simulink model "bf_4x"  (R2013a)
settings: Solver=VariableStepDiscrete  StartTime=0.0  StopTime=1000  RelTol=1e-3
undefined symbols (not defined in the file): enable, misc_lib, pfb_coeff_gen_calc
libraries: xbsIndex_r4 x6358, casper_library_misc x119, casper_library_delays x24, casper_library_multipliers x20, simulink x16, casper_library_pfbs x4, xbsReplacements_r4 x2, xps_library x1
(part 6 of 73)

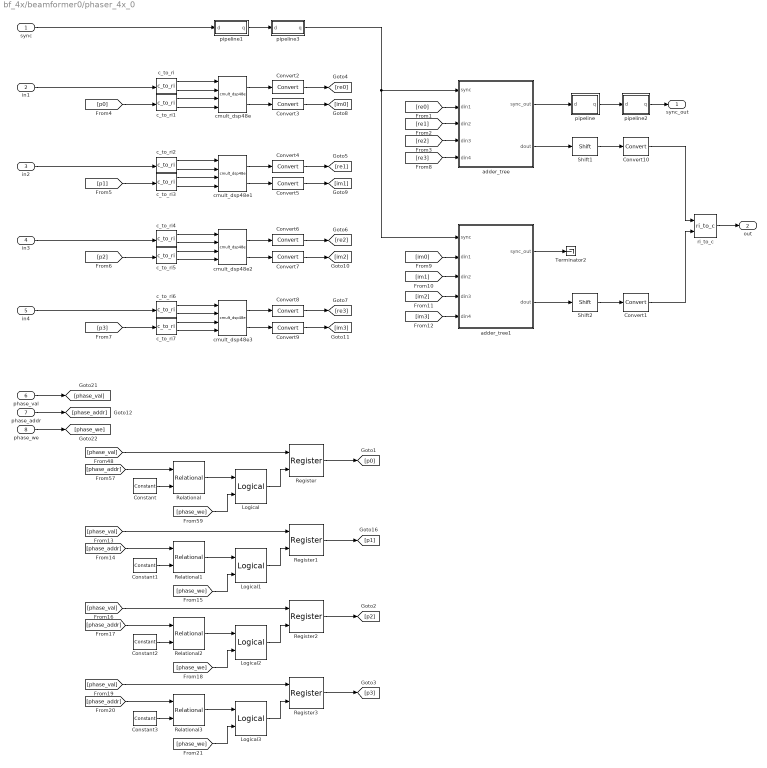
== system bf_4x/beamformer0/phaser_4x_0 ==
  sync : Inport
  in1 : Inport  Port=2
  in2 : Inport  Port=3
  in3 : Inport  Port=4
  in4 : Inport  Port=5
  phase_val : Inport  Port=6
  phase_addr : Inport  Port=7
  phase_we : Inport  Port=8
  Constant : xbsIndex_r4/Constant  const=sub_addr(1)  gui_display_data_type=Fixed-point  arith_type=Unsigned  n_bits=32  bin_pt=0  preci_type=Single  exp_width=8  frac_width=24  explicit_period=on  period=1  equ=P=C  opselect=C  inp2=PCIN>>17  opr=+  inp1=P  carry=CIN  dbl_ovrd=off  block_type=constant
  Constant1 : xbsIndex_r4/Constant  const=sub_addr(2)  gui_display_data_type=Fixed-point  arith_type=Unsigned  n_bits=32  bin_pt=0  preci_type=Single  exp_width=8  frac_width=24  explicit_period=on  period=1  equ=P=C  opselect=C  inp2=PCIN>>17  opr=+  inp1=P  carry=CIN  dbl_ovrd=off  block_type=constant
  Constant2 : xbsIndex_r4/Constant  const=sub_addr(3)  gui_display_data_type=Fixed-point  arith_type=Unsigned  n_bits=32  bin_pt=0  preci_type=Single  exp_width=8  frac_width=24  explicit_period=on  period=1  equ=P=C  opselect=C  inp2=PCIN>>17  opr=+  inp1=P  carry=CIN  dbl_ovrd=off  block_type=constant
  Constant3 : xbsIndex_r4/Constant  const=sub_addr(4)  gui_display_data_type=Fixed-point  arith_type=Unsigned  n_bits=32  bin_pt=0  preci_type=Single  exp_width=8  frac_width=24  explicit_period=on  period=1  equ=P=C  opselect=C  inp2=PCIN>>17  opr=+  inp1=P  carry=CIN  dbl_ovrd=off  block_type=constant
  Convert{1..10} (10 alike) : xbsIndex_r4/Convert  gui_display_data_type=Fixed-point  arith_type=Unsigned  n_bits=18  bin_pt=17  float_type=Single  exp_bits=8  fraction_bits=24  quantization=Truncate  overflow=Wrap  en=off  latency=2  dbl_ovrd=off  pipeline=off  block_type=convert
      settings: block_version=11.4
  Logical{,1..3} (4 alike) : xbsIndex_r4/Logical  logical_function=AND  inputs=2  en=off  latency=0  precision=Full  arith_type=Unsigned  n_bits=16  bin_pt=0  align_bp=on  dbl_ovrd=off  block_type=logical
  Register{,1..3} (4 alike) : xbsIndex_r4/Register  init=0  rst=off  en=on  dbl_ovrd=off  block_type=register
  Relational{,1..3} (4 alike) : xbsIndex_r4/Relational  mode=a=b  en=off  latency=0  dbl_ovrd=off  block_type=relational
  Shift1 : xbsIndex_r4/Shift  shift_dir=Right  shift_bits=2  en=off  latency=1  precision=Full  arith_type="Signed  (2's comp)"  n_bits=16  bin_pt=14  quantization=Truncate  overflow=Wrap  dbl_ovrd=off  block_type=shift
  Shift2 : xbsIndex_r4/Shift  shift_dir=Right  shift_bits=2  en=off  latency=1  precision=Full  arith_type="Signed  (2's comp)"  n_bits=16  bin_pt=14  quantization=Truncate  overflow=Wrap  dbl_ovrd=off  block_type=shift
  Terminator2 : Terminator
  adder_tree : Subsystem  AncestorBlock=casper_library_misc/adder_tree  mask(adder_tree){n_inputs=4, latency=1, adder_imp=Fabric, first_stage_hdl=on}
      mask prompts: n_inputs "Number of Inputs"; latency "Add Latency"; adder_imp "Adder implementation"; first_stage_hdl "Use behavioural HDL for first stage of adders"
      mask help:
      | Sums all inputs using a tree of adds and delays.
      |
      | Number of inputs: The number of inputs to the block to be summed
      | Add latency: The number of clock cycles to perform one addition (affects timing)..
      | Adder implementation: choice of fabric or DSP48E core, or behavioral HDL
      | Use behavioural HDL for first stage of adders: Causes the first stage of adders to be absorbed into DSP blocks if multipliers precede them (Virtex 5). Overrides Adder implementation
      mask init:
      | adder_tree_init(gcb, ...
      |     'n_inputs', n_inputs, ...
      |     'latency', latency, ...
      |     'adder_imp', adder_imp, ...
      |     'first_stage_hdl', first_stage_hdl);
      settings: AttributesFormatString=latency 2
      mask Help: eval('xlWeb(''http://casper.berkeley.edu/wiki/Adder_tree'')')
      mask TypeOptions adder_imp: Behavioral | Fabric | DSP48
  adder_tree1 : Subsystem  AncestorBlock=casper_library_misc/adder_tree  mask(adder_tree){n_inputs=4, latency=1, adder_imp=Fabric, first_stage_hdl=on}
      mask prompts: n_inputs "Number of Inputs"; latency "Add Latency"; adder_imp "Adder implementation"; first_stage_hdl "Use behavioural HDL for first stage of adders"
      mask help:
      | Sums all inputs using a tree of adds and delays.
      |
      | Number of inputs: The number of inputs to the block to be summed
      | Add latency: The number of clock cycles to perform one addition (affects timing)..
      | Adder implementation: choice of fabric or DSP48E core, or behavioral HDL
      | Use behavioural HDL for first stage of adders: Causes the first stage of adders to be absorbed into DSP blocks if multipliers precede them (Virtex 5). Overrides Adder implementation
      mask init:
      | adder_tree_init(gcb, ...
      |     'n_inputs', n_inputs, ...
      |     'latency', latency, ...
      |     'adder_imp', adder_imp, ...
      |     'first_stage_hdl', first_stage_hdl);
      settings: AttributesFormatString=latency 2
      mask Help: eval('xlWeb(''http://casper.berkeley.edu/wiki/Adder_tree'')')
      mask TypeOptions adder_imp: Behavioral | Fabric | DSP48
  c_to_ri{,1..7} (8 alike) : casper_library_misc/c_to_ri  n_bits=18  bin_pt=17
  cmult_dsp48e{,1..3} (4 alike) : casper_library_multipliers/cmult_dsp48e  n_bits_a=18  bin_pt_a=17  n_bits_b=18  bin_pt_b=17  conjugated=off  full_precision=on  n_bits_c=37  bin_pt_c=34  quantization=Truncate  overflow=Wrap  cast_latency=0
      settings: AttributesFormatString=|
      | 18_17 * 18_17 ==> 37_34
      | Latency=4
  pipeline : Subsystem  AncestorBlock=casper_library_delays/pipeline  mask(pipeline){latency=2}
      mask help:
      | An explicitly laid-out delay line to avoid mapping to SRL16s
      | for use in pipelining to help achieve timing closure.
      mask init:
      | pipeline_init(gcb,'latency',latency);
      settings: AttributesFormatString=Latency = %<latency>
      mask Display:
      | port_label('input', 1, 'd');
      | port_label('output', 1, 'q');
      | disp(['Z^-', num2str(latency)]);
  pipeline1 : Subsystem  AncestorBlock=casper_library_delays/pipeline  mask(pipeline){latency=4}
      mask help:
      | An explicitly laid-out delay line to avoid mapping to SRL16s
      | for use in pipelining to help achieve timing closure.
      mask init:
      | pipeline_init(gcb,'latency',latency);
      settings: AttributesFormatString=Latency = %<latency>
      mask Display:
      | port_label('input', 1, 'd');
      | port_label('output', 1, 'q');
      | disp(['Z^-', num2str(latency)]);
  pipeline2 : Subsystem  AncestorBlock=casper_library_delays/pipeline  mask(pipeline){latency=2}
      mask help:
      | An explicitly laid-out delay line to avoid mapping to SRL16s
      | for use in pipelining to help achieve timing closure.
      mask init:
      | pipeline_init(gcb,'latency',latency);
      settings: AttributesFormatString=Latency = %<latency>
      mask Display:
      | port_label('input', 1, 'd');
      | port_label('output', 1, 'q');
      | disp(['Z^-', num2str(latency)]);
  pipeline3 : Subsystem  AncestorBlock=casper_library_delays/pipeline  mask(pipeline){latency=2}
      mask help:
      | An explicitly laid-out delay line to avoid mapping to SRL16s
      | for use in pipelining to help achieve timing closure.
      mask init:
      | pipeline_init(gcb,'latency',latency);
      settings: AttributesFormatString=Latency = %<latency>
      mask Display:
      | port_label('input', 1, 'd');
      | port_label('output', 1, 'q');
      | disp(['Z^-', num2str(latency)]);
  ri_to_c : casper_library_misc/ri_to_c
  sync_out : Outport
  out : Outport  Port=2
  wires:
  phase_addr/1 -> [phase_addr]
  phase_we/1 -> [phase_we]
  [p1] -> c_to_ri3/1
  phase_val/1 -> [phase_val]
  c_to_ri3/1 -> cmult_dsp48e1/3
  Convert7/1 -> [im2]
  c_to_ri5/2 -> cmult_dsp48e2/4
  c_to_ri4/1 -> cmult_dsp48e2/1
  cmult_dsp48e2/2 -> Convert7/1
  Convert6/1 -> [re2]
  cmult_dsp48e2/1 -> Convert6/1
  [p2] -> c_to_ri5/1
  in3/1 -> c_to_ri4/1
  c_to_ri4/2 -> cmult_dsp48e2/2
  c_to_ri5/1 -> cmult_dsp48e2/3
  Convert9/1 -> [im3]
  c_to_ri7/2 -> cmult_dsp48e3/4
  c_to_ri6/1 -> cmult_dsp48e3/1
  cmult_dsp48e3/2 -> Convert9/1
  Convert8/1 -> [re3]
  cmult_dsp48e3/1 -> Convert8/1
  [p3] -> c_to_ri7/1
  in4/1 -> c_to_ri6/1
  c_to_ri6/2 -> cmult_dsp48e3/2
  c_to_ri7/1 -> cmult_dsp48e3/3
  sync/1 -> pipeline1/1(d)
  pipeline1/1(q) -> pipeline3/1(d)
  Convert3/1 -> [im0]
  c_to_ri1/2 -> cmult_dsp48e/4
  c_to_ri/1 -> cmult_dsp48e/1
  cmult_dsp48e/2 -> Convert3/1
  Convert2/1 -> [re0]
  cmult_dsp48e/1 -> Convert2/1
  [p0] -> c_to_ri1/1
  in1/1 -> c_to_ri/1
  c_to_ri/2 -> cmult_dsp48e/2
  c_to_ri1/1 -> cmult_dsp48e/3
  Convert5/1 -> [im1]
  c_to_ri3/2 -> cmult_dsp48e1/4
  c_to_ri2/1 -> cmult_dsp48e1/1
  cmult_dsp48e1/2 -> Convert5/1
  Convert4/1 -> [re1]
  cmult_dsp48e1/1 -> Convert4/1
  in2/1 -> c_to_ri2/1
  c_to_ri2/2 -> cmult_dsp48e1/2
  pipeline3/1(q) -> adder_tree1/1(sync), adder_tree/1(sync)
  adder_tree/2(dout) -> Shift1/1
  adder_tree1/2(dout) -> Shift2/1
  adder_tree/1(sync_out) -> pipeline/1(d)
  [re3] -> adder_tree/5(din4)
  [re2] -> adder_tree/4(din3)
  [re1] -> adder_tree/3(din2)
  [re0] -> adder_tree/2(din1)
  [im0] -> adder_tree1/2(din1)
  [im1] -> adder_tree1/3(din2)
  [im3] -> adder_tree1/5(din4)
  [im2] -> adder_tree1/4(din3)
  adder_tree1/1(sync_out) -> Terminator2/1
  Logical/1 -> Register/2
  Register/1 -> [p0]
  Constant/1 -> Relational/2
  Relational/1 -> Logical/1
  [phase_val] -> Register/1
  [phase_addr] -> Relational/1
  [phase_we] -> Logical/2
  Logical1/1 -> Register1/2
  Register1/1 -> [p1]
  Constant1/1 -> Relational1/2
  Relational1/1 -> Logical1/1
  [phase_val] -> Register1/1
  [phase_addr] -> Relational1/1
  [phase_we] -> Logical1/2
  Logical2/1 -> Register2/2
  Register2/1 -> [p2]
  Constant2/1 -> Relational2/2
  Relational2/1 -> Logical2/1
  [phase_val] -> Register2/1
  [phase_addr] -> Relational2/1
  [phase_we] -> Logical2/2
  Logical3/1 -> Register3/2
  Register3/1 -> [p3]
  Constant3/1 -> Relational3/2
  Relational3/1 -> Logical3/1
  [phase_val] -> Register3/1
  [phase_addr] -> Relational3/1
  [phase_we] -> Logical3/2
  pipeline/1(q) -> pipeline2/1(d)
  Shift1/1 -> Convert10/1
  Shift2/1 -> Convert1/1
  Convert1/1 -> ri_to_c/2
  Convert10/1 -> ri_to_c/1
  pipeline2/1(q) -> sync_out/1
  ri_to_c/1 -> out/1

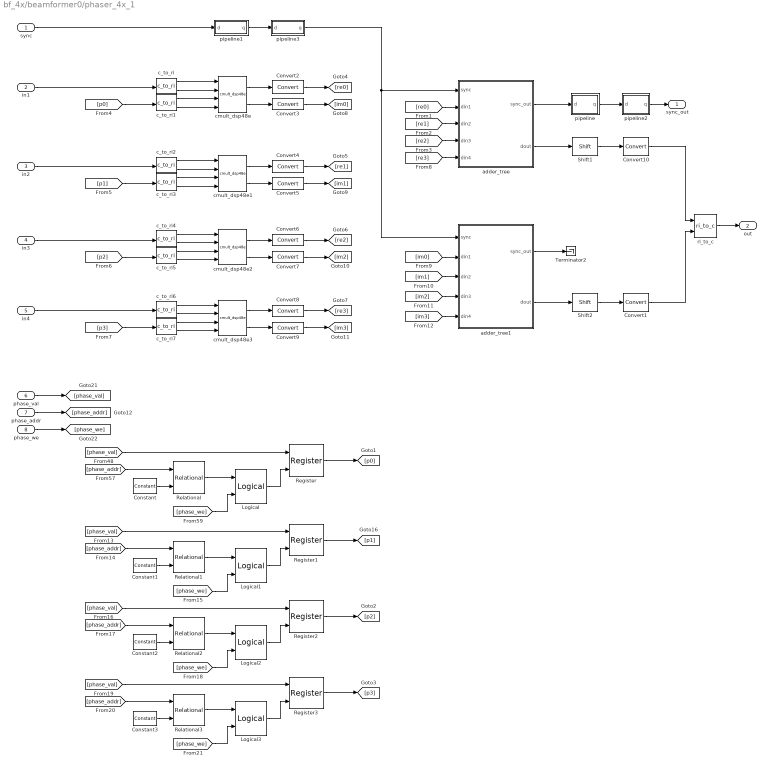
== system bf_4x/beamformer0/phaser_4x_1 ==
  sync : Inport
  in1 : Inport  Port=2
  in2 : Inport  Port=3
  in3 : Inport  Port=4
  in4 : Inport  Port=5
  phase_val : Inport  Port=6
  phase_addr : Inport  Port=7
  phase_we : Inport  Port=8
  Constant : xbsIndex_r4/Constant  const=sub_addr(1)  gui_display_data_type=Fixed-point  arith_type=Unsigned  n_bits=32  bin_pt=0  preci_type=Single  exp_width=8  frac_width=24  explicit_period=on  period=1  equ=P=C  opselect=C  inp2=PCIN>>17  opr=+  inp1=P  carry=CIN  dbl_ovrd=off  block_type=constant
  Constant1 : xbsIndex_r4/Constant  const=sub_addr(2)  gui_display_data_type=Fixed-point  arith_type=Unsigned  n_bits=32  bin_pt=0  preci_type=Single  exp_width=8  frac_width=24  explicit_period=on  period=1  equ=P=C  opselect=C  inp2=PCIN>>17  opr=+  inp1=P  carry=CIN  dbl_ovrd=off  block_type=constant
  Constant2 : xbsIndex_r4/Constant  const=sub_addr(3)  gui_display_data_type=Fixed-point  arith_type=Unsigned  n_bits=32  bin_pt=0  preci_type=Single  exp_width=8  frac_width=24  explicit_period=on  period=1  equ=P=C  opselect=C  inp2=PCIN>>17  opr=+  inp1=P  carry=CIN  dbl_ovrd=off  block_type=constant
  Constant3 : xbsIndex_r4/Constant  const=sub_addr(4)  gui_display_data_type=Fixed-point  arith_type=Unsigned  n_bits=32  bin_pt=0  preci_type=Single  exp_width=8  frac_width=24  explicit_period=on  period=1  equ=P=C  opselect=C  inp2=PCIN>>17  opr=+  inp1=P  carry=CIN  dbl_ovrd=off  block_type=constant
  Convert{1..10} (10 alike) : xbsIndex_r4/Convert  gui_display_data_type=Fixed-point  arith_type=Unsigned  n_bits=18  bin_pt=17  float_type=Single  exp_bits=8  fraction_bits=24  quantization=Truncate  overflow=Wrap  en=off  latency=2  dbl_ovrd=off  pipeline=off  block_type=convert
      settings: block_version=11.4
  Logical{,1..3} (4 alike) : xbsIndex_r4/Logical  logical_function=AND  inputs=2  en=off  latency=0  precision=Full  arith_type=Unsigned  n_bits=16  bin_pt=0  align_bp=on  dbl_ovrd=off  block_type=logical
  Register{,1..3} (4 alike) : xbsIndex_r4/Register  init=0  rst=off  en=on  dbl_ovrd=off  block_type=register
  Relational{,1..3} (4 alike) : xbsIndex_r4/Relational  mode=a=b  en=off  latency=0  dbl_ovrd=off  block_type=relational
  Shift1 : xbsIndex_r4/Shift  shift_dir=Right  shift_bits=2  en=off  latency=1  precision=Full  arith_type="Signed  (2's comp)"  n_bits=16  bin_pt=14  quantization=Truncate  overflow=Wrap  dbl_ovrd=off  block_type=shift
  Shift2 : xbsIndex_r4/Shift  shift_dir=Right  shift_bits=2  en=off  latency=1  precision=Full  arith_type="Signed  (2's comp)"  n_bits=16  bin_pt=14  quantization=Truncate  overflow=Wrap  dbl_ovrd=off  block_type=shift
  Terminator2 : Terminator
  adder_tree : Subsystem  AncestorBlock=casper_library_misc/adder_tree  mask(adder_tree){n_inputs=4, latency=1, adder_imp=Fabric, first_stage_hdl=on}
      mask prompts: n_inputs "Number of Inputs"; latency "Add Latency"; adder_imp "Adder implementation"; first_stage_hdl "Use behavioural HDL for first stage of adders"
      mask help:
      | Sums all inputs using a tree of adds and delays.
      |
      | Number of inputs: The number of inputs to the block to be summed
      | Add latency: The number of clock cycles to perform one addition (affects timing)..
      | Adder implementation: choice of fabric or DSP48E core, or behavioral HDL
      | Use behavioural HDL for first stage of adders: Causes the first stage of adders to be absorbed into DSP blocks if multipliers precede them (Virtex 5). Overrides Adder implementation
      mask init:
      | adder_tree_init(gcb, ...
      |     'n_inputs', n_inputs, ...
      |     'latency', latency, ...
      |     'adder_imp', adder_imp, ...
      |     'first_stage_hdl', first_stage_hdl);
      settings: AttributesFormatString=latency 2
      mask Help: eval('xlWeb(''http://casper.berkeley.edu/wiki/Adder_tree'')')
      mask TypeOptions adder_imp: Behavioral | Fabric | DSP48
  adder_tree1 : Subsystem  AncestorBlock=casper_library_misc/adder_tree  mask(adder_tree){n_inputs=4, latency=1, adder_imp=Fabric, first_stage_hdl=on}
      mask prompts: n_inputs "Number of Inputs"; latency "Add Latency"; adder_imp "Adder implementation"; first_stage_hdl "Use behavioural HDL for first stage of adders"
      mask help:
      | Sums all inputs using a tree of adds and delays.
      |
      | Number of inputs: The number of inputs to the block to be summed
      | Add latency: The number of clock cycles to perform one addition (affects timing)..
      | Adder implementation: choice of fabric or DSP48E core, or behavioral HDL
      | Use behavioural HDL for first stage of adders: Causes the first stage of adders to be absorbed into DSP blocks if multipliers precede them (Virtex 5). Overrides Adder implementation
      mask init:
      | adder_tree_init(gcb, ...
      |     'n_inputs', n_inputs, ...
      |     'latency', latency, ...
      |     'adder_imp', adder_imp, ...
      |     'first_stage_hdl', first_stage_hdl);
      settings: AttributesFormatString=latency 2
      mask Help: eval('xlWeb(''http://casper.berkeley.edu/wiki/Adder_tree'')')
      mask TypeOptions adder_imp: Behavioral | Fabric | DSP48
  c_to_ri{,1..7} (8 alike) : casper_library_misc/c_to_ri  n_bits=18  bin_pt=17
  cmult_dsp48e{,1..3} (4 alike) : casper_library_multipliers/cmult_dsp48e  n_bits_a=18  bin_pt_a=17  n_bits_b=18  bin_pt_b=17  conjugated=off  full_precision=on  n_bits_c=37  bin_pt_c=34  quantization=Truncate  overflow=Wrap  cast_latency=0
      settings: AttributesFormatString=|
      | 18_17 * 18_17 ==> 37_34
      | Latency=4
  pipeline : Subsystem  AncestorBlock=casper_library_delays/pipeline  mask(pipeline){latency=2}
      mask help:
      | An explicitly laid-out delay line to avoid mapping to SRL16s
      | for use in pipelining to help achieve timing closure.
      mask init:
      | pipeline_init(gcb,'latency',latency);
      settings: AttributesFormatString=Latency = %<latency>
      mask Display:
      | port_label('input', 1, 'd');
      | port_label('output', 1, 'q');
      | disp(['Z^-', num2str(latency)]);
  pipeline1 : Subsystem  AncestorBlock=casper_library_delays/pipeline  mask(pipeline){latency=4}
      mask help:
      | An explicitly laid-out delay line to avoid mapping to SRL16s
      | for use in pipelining to help achieve timing closure.
      mask init:
      | pipeline_init(gcb,'latency',latency);
      settings: AttributesFormatString=Latency = %<latency>
      mask Display:
      | port_label('input', 1, 'd');
      | port_label('output', 1, 'q');
      | disp(['Z^-', num2str(latency)]);
  pipeline2 : Subsystem  AncestorBlock=casper_library_delays/pipeline  mask(pipeline){latency=2}
      mask help:
      | An explicitly laid-out delay line to avoid mapping to SRL16s
      | for use in pipelining to help achieve timing closure.
      mask init:
      | pipeline_init(gcb,'latency',latency);
      settings: AttributesFormatString=Latency = %<latency>
      mask Display:
      | port_label('input', 1, 'd');
      | port_label('output', 1, 'q');
      | disp(['Z^-', num2str(latency)]);
  pipeline3 : Subsystem  AncestorBlock=casper_library_delays/pipeline  mask(pipeline){latency=2}
      mask help:
      | An explicitly laid-out delay line to avoid mapping to SRL16s
      | for use in pipelining to help achieve timing closure.
      mask init:
      | pipeline_init(gcb,'latency',latency);
      settings: AttributesFormatString=Latency = %<latency>
      mask Display:
      | port_label('input', 1, 'd');
      | port_label('output', 1, 'q');
      | disp(['Z^-', num2str(latency)]);
  ri_to_c : casper_library_misc/ri_to_c
  sync_out : Outport
  out : Outport  Port=2
  wires:
  ri_to_c/1 -> out/1
  pipeline2/1(q) -> sync_out/1
  Convert10/1 -> ri_to_c/1
  Convert1/1 -> ri_to_c/2
  Shift2/1 -> Convert1/1
  Shift1/1 -> Convert10/1
  pipeline/1(q) -> pipeline2/1(d)
  [phase_we] -> Logical3/2
  [phase_addr] -> Relational3/1
  [phase_val] -> Register3/1
  Relational3/1 -> Logical3/1
  Constant3/1 -> Relational3/2
  Register3/1 -> [p3]
  Logical3/1 -> Register3/2
  [phase_we] -> Logical2/2
  [phase_addr] -> Relational2/1
  [phase_val] -> Register2/1
  Relational2/1 -> Logical2/1
  Constant2/1 -> Relational2/2
  Register2/1 -> [p2]
  Logical2/1 -> Register2/2
  [phase_we] -> Logical1/2
  [phase_addr] -> Relational1/1
  [phase_val] -> Register1/1
  Relational1/1 -> Logical1/1
  Constant1/1 -> Relational1/2
  Register1/1 -> [p1]
  Logical1/1 -> Register1/2
  [phase_we] -> Logical/2
  [phase_addr] -> Relational/1
  [phase_val] -> Register/1
  Relational/1 -> Logical/1
  Constant/1 -> Relational/2
  Register/1 -> [p0]
  Logical/1 -> Register/2
  adder_tree1/1(sync_out) -> Terminator2/1
  [im2] -> adder_tree1/4(din3)
  [im3] -> adder_tree1/5(din4)
  [im1] -> adder_tree1/3(din2)
  [im0] -> adder_tree1/2(din1)
  [re0] -> adder_tree/2(din1)
  [re1] -> adder_tree/3(din2)
  [re2] -> adder_tree/4(din3)
  [re3] -> adder_tree/5(din4)
  adder_tree/1(sync_out) -> pipeline/1(d)
  adder_tree1/2(dout) -> Shift2/1
  adder_tree/2(dout) -> Shift1/1
  pipeline3/1(q) -> adder_tree/1(sync), adder_tree1/1(sync)
  c_to_ri2/2 -> cmult_dsp48e1/2
  in2/1 -> c_to_ri2/1
  cmult_dsp48e1/1 -> Convert4/1
  Convert4/1 -> [re1]
  cmult_dsp48e1/2 -> Convert5/1
  c_to_ri2/1 -> cmult_dsp48e1/1
  c_to_ri3/2 -> cmult_dsp48e1/4
  Convert5/1 -> [im1]
  c_to_ri1/1 -> cmult_dsp48e/3
  c_to_ri/2 -> cmult_dsp48e/2
  in1/1 -> c_to_ri/1
  [p0] -> c_to_ri1/1
  cmult_dsp48e/1 -> Convert2/1
  Convert2/1 -> [re0]
  cmult_dsp48e/2 -> Convert3/1
  c_to_ri/1 -> cmult_dsp48e/1
  c_to_ri1/2 -> cmult_dsp48e/4
  Convert3/1 -> [im0]
  pipeline1/1(q) -> pipeline3/1(d)
  sync/1 -> pipeline1/1(d)
  c_to_ri7/1 -> cmult_dsp48e3/3
  c_to_ri6/2 -> cmult_dsp48e3/2
  in4/1 -> c_to_ri6/1
  [p3] -> c_to_ri7/1
  cmult_dsp48e3/1 -> Convert8/1
  Convert8/1 -> [re3]
  cmult_dsp48e3/2 -> Convert9/1
  c_to_ri6/1 -> cmult_dsp48e3/1
  c_to_ri7/2 -> cmult_dsp48e3/4
  Convert9/1 -> [im3]
  c_to_ri5/1 -> cmult_dsp48e2/3
  c_to_ri4/2 -> cmult_dsp48e2/2
  in3/1 -> c_to_ri4/1
  [p2] -> c_to_ri5/1
  cmult_dsp48e2/1 -> Convert6/1
  Convert6/1 -> [re2]
  cmult_dsp48e2/2 -> Convert7/1
  c_to_ri4/1 -> cmult_dsp48e2/1
  c_to_ri5/2 -> cmult_dsp48e2/4
  Convert7/1 -> [im2]
  c_to_ri3/1 -> cmult_dsp48e1/3
  phase_val/1 -> [phase_val]
  [p1] -> c_to_ri3/1
  phase_we/1 -> [phase_we]
  phase_addr/1 -> [phase_addr]

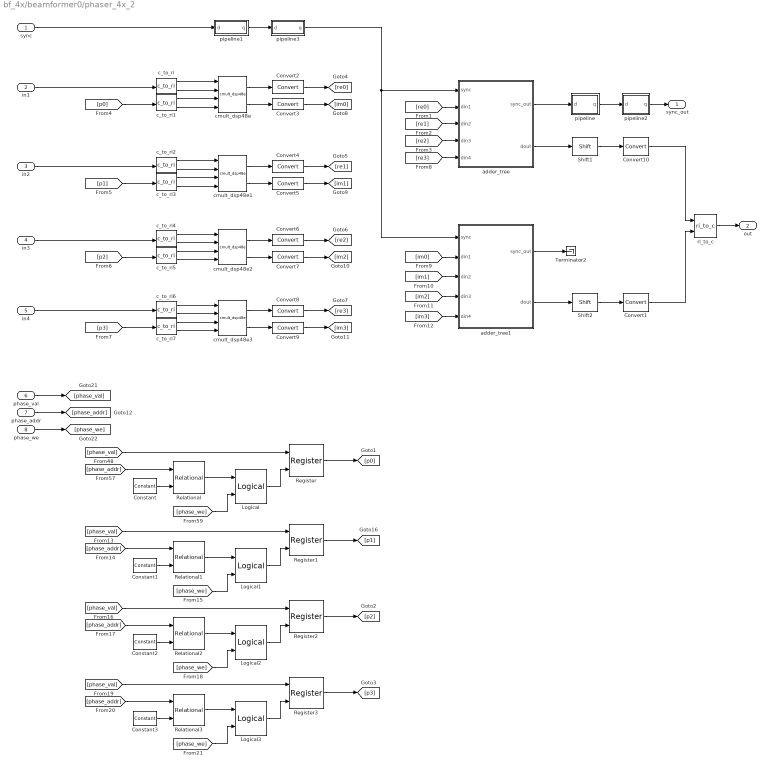
== system bf_4x/beamformer0/phaser_4x_2 ==
  sync : Inport
  in1 : Inport  Port=2
  in2 : Inport  Port=3
  in3 : Inport  Port=4
  in4 : Inport  Port=5
  phase_val : Inport  Port=6
  phase_addr : Inport  Port=7
  phase_we : Inport  Port=8
  Constant : xbsIndex_r4/Constant  const=sub_addr(1)  gui_display_data_type=Fixed-point  arith_type=Unsigned  n_bits=32  bin_pt=0  preci_type=Single  exp_width=8  frac_width=24  explicit_period=on  period=1  equ=P=C  opselect=C  inp2=PCIN>>17  opr=+  inp1=P  carry=CIN  dbl_ovrd=off  block_type=constant
  Constant1 : xbsIndex_r4/Constant  const=sub_addr(2)  gui_display_data_type=Fixed-point  arith_type=Unsigned  n_bits=32  bin_pt=0  preci_type=Single  exp_width=8  frac_width=24  explicit_period=on  period=1  equ=P=C  opselect=C  inp2=PCIN>>17  opr=+  inp1=P  carry=CIN  dbl_ovrd=off  block_type=constant
  Constant2 : xbsIndex_r4/Constant  const=sub_addr(3)  gui_display_data_type=Fixed-point  arith_type=Unsigned  n_bits=32  bin_pt=0  preci_type=Single  exp_width=8  frac_width=24  explicit_period=on  period=1  equ=P=C  opselect=C  inp2=PCIN>>17  opr=+  inp1=P  carry=CIN  dbl_ovrd=off  block_type=constant
  Constant3 : xbsIndex_r4/Constant  const=sub_addr(4)  gui_display_data_type=Fixed-point  arith_type=Unsigned  n_bits=32  bin_pt=0  preci_type=Single  exp_width=8  frac_width=24  explicit_period=on  period=1  equ=P=C  opselect=C  inp2=PCIN>>17  opr=+  inp1=P  carry=CIN  dbl_ovrd=off  block_type=constant
  Convert{1..10} (10 alike) : xbsIndex_r4/Convert  gui_display_data_type=Fixed-point  arith_type=Unsigned  n_bits=18  bin_pt=17  float_type=Single  exp_bits=8  fraction_bits=24  quantization=Truncate  overflow=Wrap  en=off  latency=2  dbl_ovrd=off  pipeline=off  block_type=convert
      settings: block_version=11.4
  Logical{,1..3} (4 alike) : xbsIndex_r4/Logical  logical_function=AND  inputs=2  en=off  latency=0  precision=Full  arith_type=Unsigned  n_bits=16  bin_pt=0  align_bp=on  dbl_ovrd=off  block_type=logical
  Register{,1..3} (4 alike) : xbsIndex_r4/Register  init=0  rst=off  en=on  dbl_ovrd=off  block_type=register
  Relational{,1..3} (4 alike) : xbsIndex_r4/Relational  mode=a=b  en=off  latency=0  dbl_ovrd=off  block_type=relational
  Shift1 : xbsIndex_r4/Shift  shift_dir=Right  shift_bits=2  en=off  latency=1  precision=Full  arith_type="Signed  (2's comp)"  n_bits=16  bin_pt=14  quantization=Truncate  overflow=Wrap  dbl_ovrd=off  block_type=shift
  Shift2 : xbsIndex_r4/Shift  shift_dir=Right  shift_bits=2  en=off  latency=1  precision=Full  arith_type="Signed  (2's comp)"  n_bits=16  bin_pt=14  quantization=Truncate  overflow=Wrap  dbl_ovrd=off  block_type=shift
  Terminator2 : Terminator
  adder_tree : Subsystem  AncestorBlock=casper_library_misc/adder_tree  mask(adder_tree){n_inputs=4, latency=1, adder_imp=Fabric, first_stage_hdl=on}
      mask prompts: n_inputs "Number of Inputs"; latency "Add Latency"; adder_imp "Adder implementation"; first_stage_hdl "Use behavioural HDL for first stage of adders"
      mask help:
      | Sums all inputs using a tree of adds and delays.
      |
      | Number of inputs: The number of inputs to the block to be summed
      | Add latency: The number of clock cycles to perform one addition (affects timing)..
      | Adder implementation: choice of fabric or DSP48E core, or behavioral HDL
      | Use behavioural HDL for first stage of adders: Causes the first stage of adders to be absorbed into DSP blocks if multipliers precede them (Virtex 5). Overrides Adder implementation
      mask init:
      | adder_tree_init(gcb, ...
      |     'n_inputs', n_inputs, ...
      |     'latency', latency, ...
      |     'adder_imp', adder_imp, ...
      |     'first_stage_hdl', first_stage_hdl);
      settings: AttributesFormatString=latency 2
      mask Help: eval('xlWeb(''http://casper.berkeley.edu/wiki/Adder_tree'')')
      mask TypeOptions adder_imp: Behavioral | Fabric | DSP48
  adder_tree1 : Subsystem  AncestorBlock=casper_library_misc/adder_tree  mask(adder_tree){n_inputs=4, latency=1, adder_imp=Fabric, first_stage_hdl=on}
      mask prompts: n_inputs "Number of Inputs"; latency "Add Latency"; adder_imp "Adder implementation"; first_stage_hdl "Use behavioural HDL for first stage of adders"
      mask help:
      | Sums all inputs using a tree of adds and delays.
      |
      | Number of inputs: The number of inputs to the block to be summed
      | Add latency: The number of clock cycles to perform one addition (affects timing)..
      | Adder implementation: choice of fabric or DSP48E core, or behavioral HDL
      | Use behavioural HDL for first stage of adders: Causes the first stage of adders to be absorbed into DSP blocks if multipliers precede them (Virtex 5). Overrides Adder implementation
      mask init:
      | adder_tree_init(gcb, ...
      |     'n_inputs', n_inputs, ...
      |     'latency', latency, ...
      |     'adder_imp', adder_imp, ...
      |     'first_stage_hdl', first_stage_hdl);
      settings: AttributesFormatString=latency 2
      mask Help: eval('xlWeb(''http://casper.berkeley.edu/wiki/Adder_tree'')')
      mask TypeOptions adder_imp: Behavioral | Fabric | DSP48
  c_to_ri{,1..7} (8 alike) : casper_library_misc/c_to_ri  n_bits=18  bin_pt=17
  cmult_dsp48e{,1..3} (4 alike) : casper_library_multipliers/cmult_dsp48e  n_bits_a=18  bin_pt_a=17  n_bits_b=18  bin_pt_b=17  conjugated=off  full_precision=on  n_bits_c=37  bin_pt_c=34  quantization=Truncate  overflow=Wrap  cast_latency=0
      settings: AttributesFormatString=|
      | 18_17 * 18_17 ==> 37_34
      | Latency=4
  pipeline : Subsystem  AncestorBlock=casper_library_delays/pipeline  mask(pipeline){latency=2}
      mask help:
      | An explicitly laid-out delay line to avoid mapping to SRL16s
      | for use in pipelining to help achieve timing closure.
      mask init:
      | pipeline_init(gcb,'latency',latency);
      settings: AttributesFormatString=Latency = %<latency>
      mask Display:
      | port_label('input', 1, 'd');
      | port_label('output', 1, 'q');
      | disp(['Z^-', num2str(latency)]);
  pipeline1 : Subsystem  AncestorBlock=casper_library_delays/pipeline  mask(pipeline){latency=4}
      mask help:
      | An explicitly laid-out delay line to avoid mapping to SRL16s
      | for use in pipelining to help achieve timing closure.
      mask init:
      | pipeline_init(gcb,'latency',latency);
      settings: AttributesFormatString=Latency = %<latency>
      mask Display:
      | port_label('input', 1, 'd');
      | port_label('output', 1, 'q');
      | disp(['Z^-', num2str(latency)]);
  pipeline2 : Subsystem  AncestorBlock=casper_library_delays/pipeline  mask(pipeline){latency=2}
      mask help:
      | An explicitly laid-out delay line to avoid mapping to SRL16s
      | for use in pipelining to help achieve timing closure.
      mask init:
      | pipeline_init(gcb,'latency',latency);
      settings: AttributesFormatString=Latency = %<latency>
      mask Display:
      | port_label('input', 1, 'd');
      | port_label('output', 1, 'q');
      | disp(['Z^-', num2str(latency)]);
  pipeline3 : Subsystem  AncestorBlock=casper_library_delays/pipeline  mask(pipeline){latency=2}
      mask help:
      | An explicitly laid-out delay line to avoid mapping to SRL16s
      | for use in pipelining to help achieve timing closure.
      mask init:
      | pipeline_init(gcb,'latency',latency);
      settings: AttributesFormatString=Latency = %<latency>
      mask Display:
      | port_label('input', 1, 'd');
      | port_label('output', 1, 'q');
      | disp(['Z^-', num2str(latency)]);
  ri_to_c : casper_library_misc/ri_to_c
  sync_out : Outport
  out : Outport  Port=2
  wires:
  phase_addr/1 -> [phase_addr]
  phase_we/1 -> [phase_we]
  [p1] -> c_to_ri3/1
  phase_val/1 -> [phase_val]
  c_to_ri3/1 -> cmult_dsp48e1/3
  Convert7/1 -> [im2]
  c_to_ri5/2 -> cmult_dsp48e2/4
  c_to_ri4/1 -> cmult_dsp48e2/1
  cmult_dsp48e2/2 -> Convert7/1
  Convert6/1 -> [re2]
  cmult_dsp48e2/1 -> Convert6/1
  [p2] -> c_to_ri5/1
  in3/1 -> c_to_ri4/1
  c_to_ri4/2 -> cmult_dsp48e2/2
  c_to_ri5/1 -> cmult_dsp48e2/3
  Convert9/1 -> [im3]
  c_to_ri7/2 -> cmult_dsp48e3/4
  c_to_ri6/1 -> cmult_dsp48e3/1
  cmult_dsp48e3/2 -> Convert9/1
  Convert8/1 -> [re3]
  cmult_dsp48e3/1 -> Convert8/1
  [p3] -> c_to_ri7/1
  in4/1 -> c_to_ri6/1
  c_to_ri6/2 -> cmult_dsp48e3/2
  c_to_ri7/1 -> cmult_dsp48e3/3
  sync/1 -> pipeline1/1(d)
  pipeline1/1(q) -> pipeline3/1(d)
  Convert3/1 -> [im0]
  c_to_ri1/2 -> cmult_dsp48e/4
  c_to_ri/1 -> cmult_dsp48e/1
  cmult_dsp48e/2 -> Convert3/1
  Convert2/1 -> [re0]
  cmult_dsp48e/1 -> Convert2/1
  [p0] -> c_to_ri1/1
  in1/1 -> c_to_ri/1
  c_to_ri/2 -> cmult_dsp48e/2
  c_to_ri1/1 -> cmult_dsp48e/3
  Convert5/1 -> [im1]
  c_to_ri3/2 -> cmult_dsp48e1/4
  c_to_ri2/1 -> cmult_dsp48e1/1
  cmult_dsp48e1/2 -> Convert5/1
  Convert4/1 -> [re1]
  cmult_dsp48e1/1 -> Convert4/1
  in2/1 -> c_to_ri2/1
  c_to_ri2/2 -> cmult_dsp48e1/2
  pipeline3/1(q) -> adder_tree1/1(sync), adder_tree/1(sync)
  adder_tree/2(dout) -> Shift1/1
  adder_tree1/2(dout) -> Shift2/1
  adder_tree/1(sync_out) -> pipeline/1(d)
  [re3] -> adder_tree/5(din4)
  [re2] -> adder_tree/4(din3)
  [re1] -> adder_tree/3(din2)
  [re0] -> adder_tree/2(din1)
  [im0] -> adder_tree1/2(din1)
  [im1] -> adder_tree1/3(din2)
  [im3] -> adder_tree1/5(din4)
  [im2] -> adder_tree1/4(din3)
  adder_tree1/1(sync_out) -> Terminator2/1
  Logical/1 -> Register/2
  Register/1 -> [p0]
  Constant/1 -> Relational/2
  Relational/1 -> Logical/1
  [phase_val] -> Register/1
  [phase_addr] -> Relational/1
  [phase_we] -> Logical/2
  Logical1/1 -> Register1/2
  Register1/1 -> [p1]
  Constant1/1 -> Relational1/2
  Relational1/1 -> Logical1/1
  [phase_val] -> Register1/1
  [phase_addr] -> Relational1/1
  [phase_we] -> Logical1/2
  Logical2/1 -> Register2/2
  Register2/1 -> [p2]
  Constant2/1 -> Relational2/2
  Relational2/1 -> Logical2/1
  [phase_val] -> Register2/1
  [phase_addr] -> Relational2/1
  [phase_we] -> Logical2/2
  Logical3/1 -> Register3/2
  Register3/1 -> [p3]
  Constant3/1 -> Relational3/2
  Relational3/1 -> Logical3/1
  [phase_val] -> Register3/1
  [phase_addr] -> Relational3/1
  [phase_we] -> Logical3/2
  pipeline/1(q) -> pipeline2/1(d)
  Shift1/1 -> Convert10/1
  Shift2/1 -> Convert1/1
  Convert1/1 -> ri_to_c/2
  Convert10/1 -> ri_to_c/1
  pipeline2/1(q) -> sync_out/1
  ri_to_c/1 -> out/1

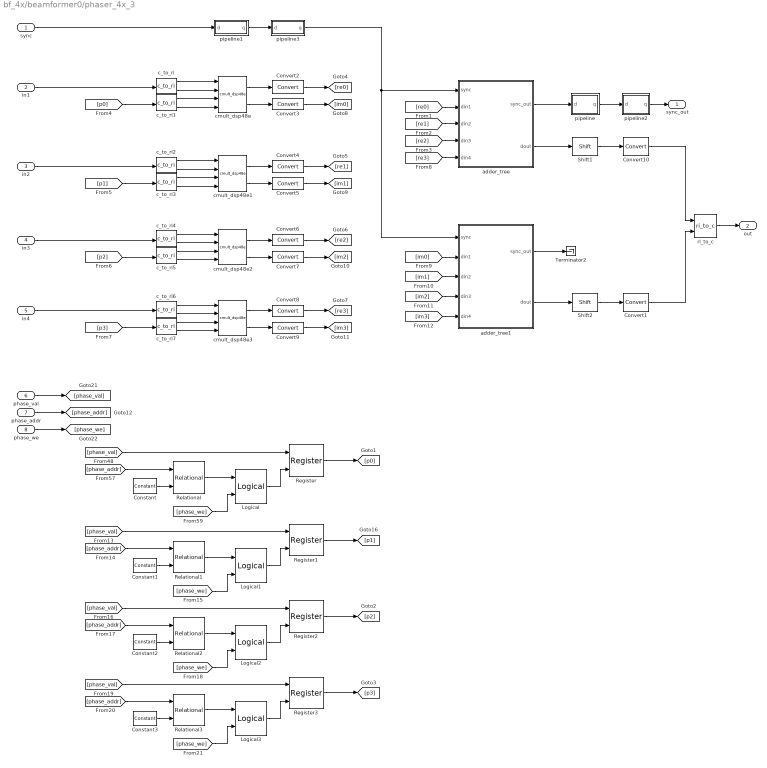
== system bf_4x/beamformer0/phaser_4x_3 ==
  sync : Inport
  in1 : Inport  Port=2
  in2 : Inport  Port=3
  in3 : Inport  Port=4
  in4 : Inport  Port=5
  phase_val : Inport  Port=6
  phase_addr : Inport  Port=7
  phase_we : Inport  Port=8
  Constant : xbsIndex_r4/Constant  const=sub_addr(1)  gui_display_data_type=Fixed-point  arith_type=Unsigned  n_bits=32  bin_pt=0  preci_type=Single  exp_width=8  frac_width=24  explicit_period=on  period=1  equ=P=C  opselect=C  inp2=PCIN>>17  opr=+  inp1=P  carry=CIN  dbl_ovrd=off  block_type=constant
  Constant1 : xbsIndex_r4/Constant  const=sub_addr(2)  gui_display_data_type=Fixed-point  arith_type=Unsigned  n_bits=32  bin_pt=0  preci_type=Single  exp_width=8  frac_width=24  explicit_period=on  period=1  equ=P=C  opselect=C  inp2=PCIN>>17  opr=+  inp1=P  carry=CIN  dbl_ovrd=off  block_type=constant
  Constant2 : xbsIndex_r4/Constant  const=sub_addr(3)  gui_display_data_type=Fixed-point  arith_type=Unsigned  n_bits=32  bin_pt=0  preci_type=Single  exp_width=8  frac_width=24  explicit_period=on  period=1  equ=P=C  opselect=C  inp2=PCIN>>17  opr=+  inp1=P  carry=CIN  dbl_ovrd=off  block_type=constant
  Constant3 : xbsIndex_r4/Constant  const=sub_addr(4)  gui_display_data_type=Fixed-point  arith_type=Unsigned  n_bits=32  bin_pt=0  preci_type=Single  exp_width=8  frac_width=24  explicit_period=on  period=1  equ=P=C  opselect=C  inp2=PCIN>>17  opr=+  inp1=P  carry=CIN  dbl_ovrd=off  block_type=constant
  Convert{1..10} (10 alike) : xbsIndex_r4/Convert  gui_display_data_type=Fixed-point  arith_type=Unsigned  n_bits=18  bin_pt=17  float_type=Single  exp_bits=8  fraction_bits=24  quantization=Truncate  overflow=Wrap  en=off  latency=2  dbl_ovrd=off  pipeline=off  block_type=convert
      settings: block_version=11.4
  Logical{,1..3} (4 alike) : xbsIndex_r4/Logical  logical_function=AND  inputs=2  en=off  latency=0  precision=Full  arith_type=Unsigned  n_bits=16  bin_pt=0  align_bp=on  dbl_ovrd=off  block_type=logical
  Register{,1..3} (4 alike) : xbsIndex_r4/Register  init=0  rst=off  en=on  dbl_ovrd=off  block_type=register
  Relational{,1..3} (4 alike) : xbsIndex_r4/Relational  mode=a=b  en=off  latency=0  dbl_ovrd=off  block_type=relational
  Shift1 : xbsIndex_r4/Shift  shift_dir=Right  shift_bits=2  en=off  latency=1  precision=Full  arith_type="Signed  (2's comp)"  n_bits=16  bin_pt=14  quantization=Truncate  overflow=Wrap  dbl_ovrd=off  block_type=shift
  Shift2 : xbsIndex_r4/Shift  shift_dir=Right  shift_bits=2  en=off  latency=1  precision=Full  arith_type="Signed  (2's comp)"  n_bits=16  bin_pt=14  quantization=Truncate  overflow=Wrap  dbl_ovrd=off  block_type=shift
  Terminator2 : Terminator
  adder_tree : Subsystem  AncestorBlock=casper_library_misc/adder_tree  mask(adder_tree){n_inputs=4, latency=1, adder_imp=Fabric, first_stage_hdl=on}
      mask prompts: n_inputs "Number of Inputs"; latency "Add Latency"; adder_imp "Adder implementation"; first_stage_hdl "Use behavioural HDL for first stage of adders"
      mask help:
      | Sums all inputs using a tree of adds and delays.
      |
      | Number of inputs: The number of inputs to the block to be summed
      | Add latency: The number of clock cycles to perform one addition (affects timing)..
      | Adder implementation: choice of fabric or DSP48E core, or behavioral HDL
      | Use behavioural HDL for first stage of adders: Causes the first stage of adders to be absorbed into DSP blocks if multipliers precede them (Virtex 5). Overrides Adder implementation
      mask init:
      | adder_tree_init(gcb, ...
      |     'n_inputs', n_inputs, ...
      |     'latency', latency, ...
      |     'adder_imp', adder_imp, ...
      |     'first_stage_hdl', first_stage_hdl);
      settings: AttributesFormatString=latency 2
      mask Help: eval('xlWeb(''http://casper.berkeley.edu/wiki/Adder_tree'')')
      mask TypeOptions adder_imp: Behavioral | Fabric | DSP48
  adder_tree1 : Subsystem  AncestorBlock=casper_library_misc/adder_tree  mask(adder_tree){n_inputs=4, latency=1, adder_imp=Fabric, first_stage_hdl=on}
      mask prompts: n_inputs "Number of Inputs"; latency "Add Latency"; adder_imp "Adder implementation"; first_stage_hdl "Use behavioural HDL for first stage of adders"
      mask help:
      | Sums all inputs using a tree of adds and delays.
      |
      | Number of inputs: The number of inputs to the block to be summed
      | Add latency: The number of clock cycles to perform one addition (affects timing)..
      | Adder implementation: choice of fabric or DSP48E core, or behavioral HDL
      | Use behavioural HDL for first stage of adders: Causes the first stage of adders to be absorbed into DSP blocks if multipliers precede them (Virtex 5). Overrides Adder implementation
      mask init:
      | adder_tree_init(gcb, ...
      |     'n_inputs', n_inputs, ...
      |     'latency', latency, ...
      |     'adder_imp', adder_imp, ...
      |     'first_stage_hdl', first_stage_hdl);
      settings: AttributesFormatString=latency 2
      mask Help: eval('xlWeb(''http://casper.berkeley.edu/wiki/Adder_tree'')')
      mask TypeOptions adder_imp: Behavioral | Fabric | DSP48
  c_to_ri{,1..7} (8 alike) : casper_library_misc/c_to_ri  n_bits=18  bin_pt=17
  cmult_dsp48e{,1..3} (4 alike) : casper_library_multipliers/cmult_dsp48e  n_bits_a=18  bin_pt_a=17  n_bits_b=18  bin_pt_b=17  conjugated=off  full_precision=on  n_bits_c=37  bin_pt_c=34  quantization=Truncate  overflow=Wrap  cast_latency=0
      settings: AttributesFormatString=|
      | 18_17 * 18_17 ==> 37_34
      | Latency=4
  pipeline : Subsystem  AncestorBlock=casper_library_delays/pipeline  mask(pipeline){latency=2}
      mask help:
      | An explicitly laid-out delay line to avoid mapping to SRL16s
      | for use in pipelining to help achieve timing closure.
      mask init:
      | pipeline_init(gcb,'latency',latency);
      settings: AttributesFormatString=Latency = %<latency>
      mask Display:
      | port_label('input', 1, 'd');
      | port_label('output', 1, 'q');
      | disp(['Z^-', num2str(latency)]);
  pipeline1 : Subsystem  AncestorBlock=casper_library_delays/pipeline  mask(pipeline){latency=4}
      mask help:
      | An explicitly laid-out delay line to avoid mapping to SRL16s
      | for use in pipelining to help achieve timing closure.
      mask init:
      | pipeline_init(gcb,'latency',latency);
      settings: AttributesFormatString=Latency = %<latency>
      mask Display:
      | port_label('input', 1, 'd');
      | port_label('output', 1, 'q');
      | disp(['Z^-', num2str(latency)]);
  pipeline2 : Subsystem  AncestorBlock=casper_library_delays/pipeline  mask(pipeline){latency=2}
      mask help:
      | An explicitly laid-out delay line to avoid mapping to SRL16s
      | for use in pipelining to help achieve timing closure.
      mask init:
      | pipeline_init(gcb,'latency',latency);
      settings: AttributesFormatString=Latency = %<latency>
      mask Display:
      | port_label('input', 1, 'd');
      | port_label('output', 1, 'q');
      | disp(['Z^-', num2str(latency)]);
  pipeline3 : Subsystem  AncestorBlock=casper_library_delays/pipeline  mask(pipeline){latency=2}
      mask help:
      | An explicitly laid-out delay line to avoid mapping to SRL16s
      | for use in pipelining to help achieve timing closure.
      mask init:
      | pipeline_init(gcb,'latency',latency);
      settings: AttributesFormatString=Latency = %<latency>
      mask Display:
      | port_label('input', 1, 'd');
      | port_label('output', 1, 'q');
      | disp(['Z^-', num2str(latency)]);
  ri_to_c : casper_library_misc/ri_to_c
  sync_out : Outport
  out : Outport  Port=2
  wires:
  ri_to_c/1 -> out/1
  pipeline2/1(q) -> sync_out/1
  Convert10/1 -> ri_to_c/1
  Convert1/1 -> ri_to_c/2
  Shift2/1 -> Convert1/1
  Shift1/1 -> Convert10/1
  pipeline/1(q) -> pipeline2/1(d)
  [phase_we] -> Logical3/2
  [phase_addr] -> Relational3/1
  [phase_val] -> Register3/1
  Relational3/1 -> Logical3/1
  Constant3/1 -> Relational3/2
  Register3/1 -> [p3]
  Logical3/1 -> Register3/2
  [phase_we] -> Logical2/2
  [phase_addr] -> Relational2/1
  [phase_val] -> Register2/1
  Relational2/1 -> Logical2/1
  Constant2/1 -> Relational2/2
  Register2/1 -> [p2]
  Logical2/1 -> Register2/2
  [phase_we] -> Logical1/2
  [phase_addr] -> Relational1/1
  [phase_val] -> Register1/1
  Relational1/1 -> Logical1/1
  Constant1/1 -> Relational1/2
  Register1/1 -> [p1]
  Logical1/1 -> Register1/2
  [phase_we] -> Logical/2
  [phase_addr] -> Relational/1
  [phase_val] -> Register/1
  Relational/1 -> Logical/1
  Constant/1 -> Relational/2
  Register/1 -> [p0]
  Logical/1 -> Register/2
  adder_tree1/1(sync_out) -> Terminator2/1
  [im2] -> adder_tree1/4(din3)
  [im3] -> adder_tree1/5(din4)
  [im1] -> adder_tree1/3(din2)
  [im0] -> adder_tree1/2(din1)
  [re0] -> adder_tree/2(din1)
  [re1] -> adder_tree/3(din2)
  [re2] -> adder_tree/4(din3)
  [re3] -> adder_tree/5(din4)
  adder_tree/1(sync_out) -> pipeline/1(d)
  adder_tree1/2(dout) -> Shift2/1
  adder_tree/2(dout) -> Shift1/1
  pipeline3/1(q) -> adder_tree/1(sync), adder_tree1/1(sync)
  c_to_ri2/2 -> cmult_dsp48e1/2
  in2/1 -> c_to_ri2/1
  cmult_dsp48e1/1 -> Convert4/1
  Convert4/1 -> [re1]
  cmult_dsp48e1/2 -> Convert5/1
  c_to_ri2/1 -> cmult_dsp48e1/1
  c_to_ri3/2 -> cmult_dsp48e1/4
  Convert5/1 -> [im1]
  c_to_ri1/1 -> cmult_dsp48e/3
  c_to_ri/2 -> cmult_dsp48e/2
  in1/1 -> c_to_ri/1
  [p0] -> c_to_ri1/1
  cmult_dsp48e/1 -> Convert2/1
  Convert2/1 -> [re0]
  cmult_dsp48e/2 -> Convert3/1
  c_to_ri/1 -> cmult_dsp48e/1
  c_to_ri1/2 -> cmult_dsp48e/4
  Convert3/1 -> [im0]
  pipeline1/1(q) -> pipeline3/1(d)
  sync/1 -> pipeline1/1(d)
  c_to_ri7/1 -> cmult_dsp48e3/3
  c_to_ri6/2 -> cmult_dsp48e3/2
  in4/1 -> c_to_ri6/1
  [p3] -> c_to_ri7/1
  cmult_dsp48e3/1 -> Convert8/1
  Convert8/1 -> [re3]
  cmult_dsp48e3/2 -> Convert9/1
  c_to_ri6/1 -> cmult_dsp48e3/1
  c_to_ri7/2 -> cmult_dsp48e3/4
  Convert9/1 -> [im3]
  c_to_ri5/1 -> cmult_dsp48e2/3
  c_to_ri4/2 -> cmult_dsp48e2/2
  in3/1 -> c_to_ri4/1
  [p2] -> c_to_ri5/1
  cmult_dsp48e2/1 -> Convert6/1
  Convert6/1 -> [re2]
  cmult_dsp48e2/2 -> Convert7/1
  c_to_ri4/1 -> cmult_dsp48e2/1
  c_to_ri5/2 -> cmult_dsp48e2/4
  Convert7/1 -> [im2]
  c_to_ri3/1 -> cmult_dsp48e1/3
  phase_val/1 -> [phase_val]
  [p1] -> c_to_ri3/1
  phase_we/1 -> [phase_we]
  phase_addr/1 -> [phase_addr]

== system bf_4x/beamformer0/pipeline1 ==
  d : Inport
  Register0 : xbsIndex_r4/Register  init=0  rst=off  en=off  dbl_ovrd=off  block_type=register
      settings: block_version=11.4
  Register1 : xbsIndex_r4/Register  init=0  rst=off  en=off  dbl_ovrd=off  block_type=register
      settings: block_version=11.4
  q : Outport
  wires:
  Register1/1 -> q/1
  d/1 -> Register0/1
  Register0/1 -> Register1/1

== system bf_4x/beamformer0/pipeline2 ==
  d : Inport
  Register0 : xbsIndex_r4/Register  init=0  rst=off  en=off  dbl_ovrd=off  block_type=register
      settings: block_version=11.4
  Register1 : xbsIndex_r4/Register  init=0  rst=off  en=off  dbl_ovrd=off  block_type=register
      settings: block_version=11.4
  q : Outport
  wires:
  Register0/1 -> Register1/1
  d/1 -> Register0/1
  Register1/1 -> q/1
